simulink model "SMCController1"  (R2018a)
settings: Solver=VariableStepAuto  StartTime=0.0  StopTime=150  RelTol=1e-1
settings Model: Creator=varunpwr  LastModifiedBy=varunpwr

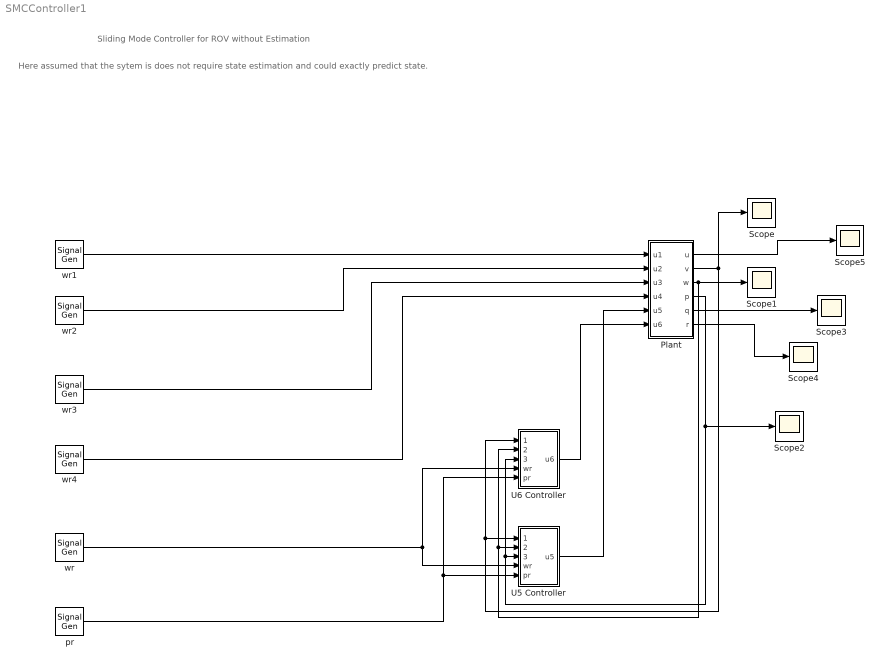
== system SMCController1 ==
  note: Here assumed that the sytem is does not require state estimation and could exactly predict state.
  note: Sliding Mode Controller for ROV without Estimation
  Plant : Subsystem
  Scope{,1..5} (6 alike) : Scope
  U5 Controller : Subsystem
  "U6 Controller " : Subsystem
  pr : SignalGenerator  Amplitude=0  Units=rad/sec
  wr : SignalGenerator  WaveForm=square  Amplitude=0.001  Units=rad/sec
  wr{1..4} (4 alike) : SignalGenerator  Amplitude=0  Units=rad/sec
  wires:
  Plant/2(v) -> Scope/1, "U6 Controller "/1("v var "), U5 Controller/1(v var)
  Plant/3(w) -> Scope1/1, "U6 Controller "/2("w var "), U5 Controller/2("w var ")
  Plant/4(p) -> Scope2/1, "U6 Controller "/3("p var "), U5 Controller/3(p var)
  wr/1 -> U5 Controller/4(wr), "U6 Controller "/4(wr)
  pr/1 -> U5 Controller/5(pr), "U6 Controller "/5(pr)
  U5 Controller/1(u5) -> Plant/5(u5)
  "U6 Controller "/1("u6 ") -> Plant/6(u6)
  wr1/1 -> Plant/1(u1)
  wr2/1 -> Plant/2(u2)
  wr3/1 -> Plant/3(u3)
  wr4/1 -> Plant/4(u4)
  Plant/5(q) -> Scope3/1
  Plant/6(r) -> Scope4/1
  Plant/1("u ") -> Scope5/1

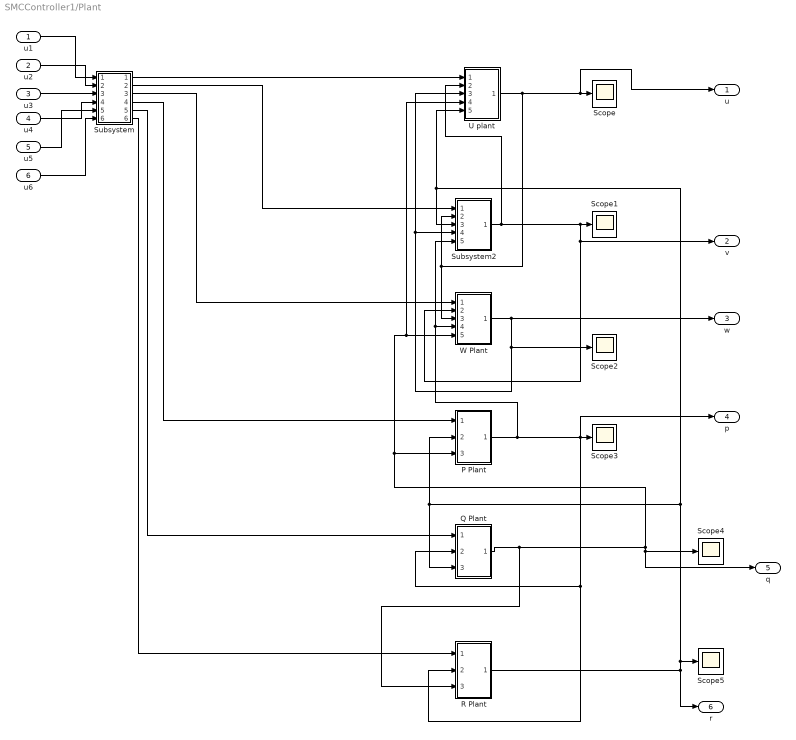
== system SMCController1/Plant ==
  u1 : Inport
  u2 : Inport  Port=2
  u3 : Inport  Port=3
  u4 : Inport  Port=4
  u5 : Inport  Port=5
  u6 : Inport  Port=6
  P Plant : Subsystem
  Q Plant : Subsystem
  "R Plant " : Subsystem
  Scope{,1..5} (6 alike) : Scope
  Subsystem : Subsystem
  Subsystem2 : Subsystem
  "U plant " : Subsystem
  "W Plant " : Subsystem
  "u " : Outport
  v : Outport  Port=2
  w : Outport  Port=3
  p : Outport  Port=4
  q : Outport  Port=5
  r : Outport  Port=6
  wires:
  Subsystem/1(Out1) -> "U plant "/1(In1)
  u2/1 -> Subsystem/2(In2)
  Subsystem/2(Out2) -> Subsystem2/1(In1)
  Subsystem/3(Out3) -> "W Plant "/1(In1)
  u1/1 -> Subsystem/1(In1)
  Q Plant/1(Out1) -> Scope4/1, q/1, P Plant/3("In3 "), "W Plant "/5(In5), "U plant "/4(In4), "R Plant "/3(In3)
  u6/1 -> Subsystem/6(In6)
  Subsystem/6(Out6) -> "R Plant "/1(In1)
  Subsystem2/1(Out1) -> "W Plant "/2(In2), v/1, Scope1/1, "U plant "/2(In2)
  u4/1 -> Subsystem/4(In4)
  "U plant "/1(Out1) -> Subsystem2/2(In2), "W Plant "/3(In3), "u "/1, Scope/1
  u5/1 -> Subsystem/5(In5)
  "R Plant "/1(Out1) -> r/1, Scope5/1, Q Plant/3(In3), P Plant/2(In2), Subsystem2/3(In3), "U plant "/5(In5)
  u3/1 -> Subsystem/3(In3)
  P Plant/1(Out1) -> "R Plant "/2(In2), Q Plant/2(In2), Scope3/1, p/1, "W Plant "/4(In4), Subsystem2/5(In5)
  Subsystem/5(Out5) -> Q Plant/1(In1)
  "W Plant "/1(Out1) -> w/1, Scope2/1, Subsystem2/4(In4), "U plant "/3(In3)
  Subsystem/4(Out4) -> P Plant/1(In1)

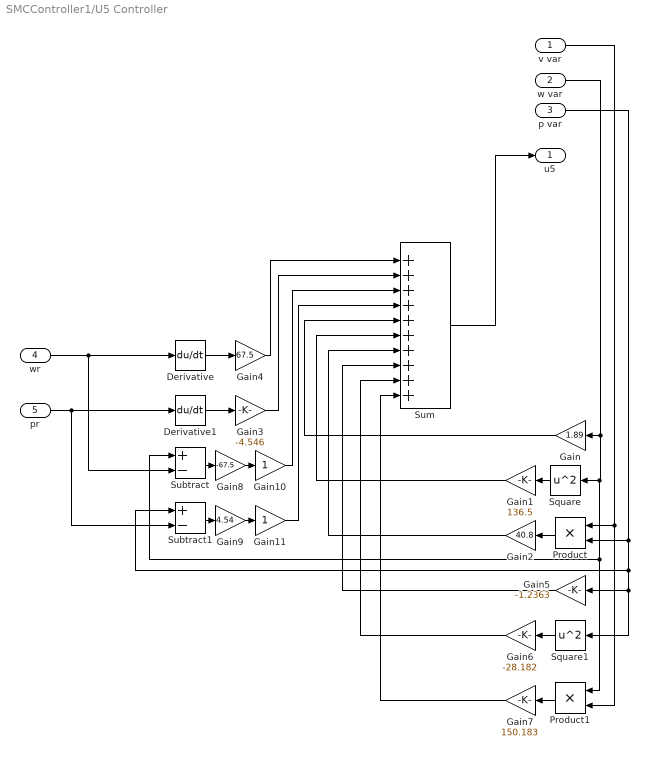
== system SMCController1/U5 Controller ==
  v var : Inport
  "w var " : Inport  Port=2
  p var : Inport  Port=3
  wr : Inport  Port=4
  pr : Inport  Port=5
  Derivative : Derivative
  Derivative1 : Derivative
  Gain : Gain  Gain=1.89
  Gain1 : Gain  Gain=136.5
  Gain10 : Gain
  Gain11 : Gain
  Gain2 : Gain  Gain=40.8
  Gain3 : Gain  Gain=-4.546
  Gain4 : Gain  Gain=67.5
  Gain5 : Gain  Gain=-1.2363
  Gain6 : Gain  Gain=-28.182
  Gain7 : Gain  Gain=150.183
  Gain8 : Gain  Gain=-67.5
  Gain9 : Gain  Gain=4.54
  Product : Product
  Product1 : Product
  Square : Math  Operator=square  SaturateOnIntegerOverflow=on
  Square1 : Math  Operator=square  SaturateOnIntegerOverflow=on
  Subtract : Sum  Inputs=+-
  Subtract1 : Sum  Inputs=+-
  Sum : Sum  Inputs=|++++++++++
  u5 : Outport
  wires:
  Square1/1 -> Gain6/1
  Subtract1/1 -> Gain9/1
  wr/1 -> Subtract/2, Derivative/1
  Gain5/1 -> Sum/8
  "w var "/1 -> Subtract/1, Product1/1, Square/1, Gain/1
  pr/1 -> Subtract1/2, Derivative1/1
  Gain/1 -> Sum/5
  Subtract/1 -> Gain8/1
  v var/1 -> Product1/2, Product/1
  Sum/1 -> u5/1
  p var/1 -> Subtract1/1, Square1/1, Gain5/1, Product/2
  Gain3/1 -> Sum/2
  Square/1 -> Gain1/1
  Gain2/1 -> Sum/7
  Product1/1 -> Gain7/1
  Gain6/1 -> Sum/9
  Gain4/1 -> Sum/1
  Product/1 -> Gain2/1
  Derivative1/1 -> Gain3/1
  Derivative/1 -> Gain4/1
  Gain7/1 -> Sum/10
  Gain1/1 -> Sum/6
  Gain8/1 -> Gain10/1
  Gain10/1 -> Sum/3
  Gain9/1 -> Gain11/1
  Gain11/1 -> Sum/4

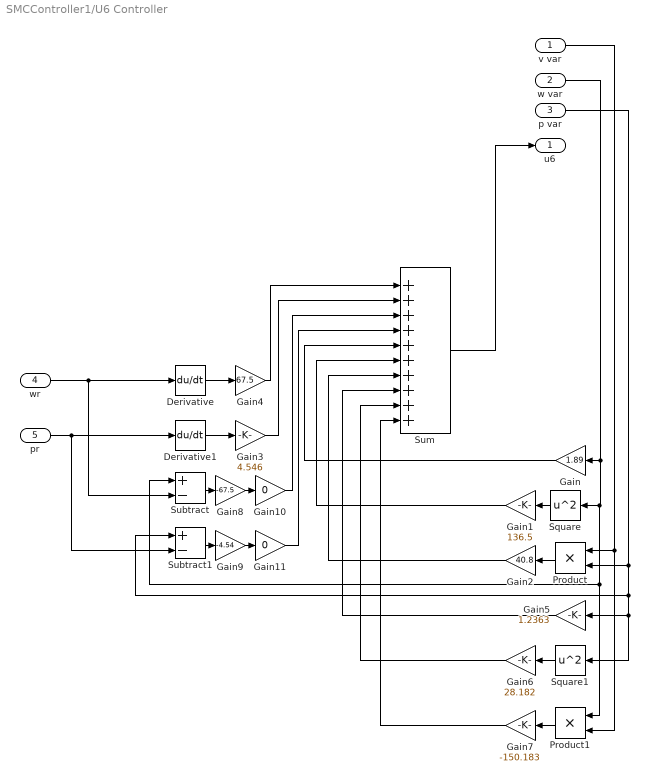
== system SMCController1/U6 Controller  ==
  "v var " : Inport
  "w var " : Inport  Port=2
  "p var " : Inport  Port=3
  wr : Inport  Port=4
  pr : Inport  Port=5
  Derivative : Derivative
  Derivative1 : Derivative
  Gain : Gain  Gain=1.89
  Gain1 : Gain  Gain=136.5
  Gain10 : Gain  Gain=0
  Gain11 : Gain  Gain=0
  Gain2 : Gain  Gain=40.8
  Gain3 : Gain  Gain=4.546
  Gain4 : Gain  Gain=67.5
  Gain5 : Gain  Gain=1.2363
  Gain6 : Gain  Gain=28.182
  Gain7 : Gain  Gain=-150.183
  Gain8 : Gain  Gain=-67.5
  Gain9 : Gain  Gain=-4.54
  Product : Product
  Product1 : Product
  Square : Math  Operator=square  SaturateOnIntegerOverflow=on
  Square1 : Math  Operator=square  SaturateOnIntegerOverflow=on
  Subtract : Sum  Inputs=+-
  Subtract1 : Sum  Inputs=+-
  Sum : Sum  Inputs=|++++++++++
  "u6 " : Outport
  wires:
  Gain1/1 -> Sum/6
  Gain7/1 -> Sum/10
  Derivative/1 -> Gain4/1
  Derivative1/1 -> Gain3/1
  Product/1 -> Gain2/1
  Gain4/1 -> Sum/1
  Gain6/1 -> Sum/9
  Product1/1 -> Gain7/1
  Gain2/1 -> Sum/7
  Square/1 -> Gain1/1
  Gain3/1 -> Sum/2
  "p var "/1 -> Product/2, Gain5/1, Square1/1, Subtract1/1
  Sum/1 -> "u6 "/1
  "v var "/1 -> Product/1, Product1/2
  Subtract/1 -> Gain8/1
  Gain/1 -> Sum/5
  pr/1 -> Derivative1/1, Subtract1/2
  "w var "/1 -> Gain/1, Square/1, Product1/1, Subtract/1
  Gain5/1 -> Sum/8
  wr/1 -> Derivative/1, Subtract/2
  Subtract1/1 -> Gain9/1
  Square1/1 -> Gain6/1
  Gain8/1 -> Gain10/1
  Gain10/1 -> Sum/3
  Gain9/1 -> Gain11/1
  Gain11/1 -> Sum/4

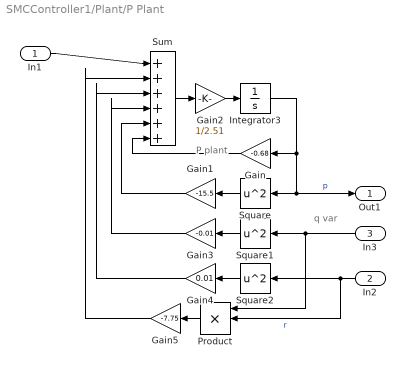
== system SMCController1/Plant/P Plant ==
  note: q var
  note: P plant
  In1 : Inport
  In2 : Inport  Port=2
  "In3 " : Inport  Port=3
  Gain : Gain  Gain=-0.68
  Gain1 : Gain  Gain=-15.5
  Gain2 : Gain  Gain=1/2.51
  Gain3 : Gain  Gain=-0.01
  Gain4 : Gain  Gain=0.01
  Gain5 : Gain  Gain=-7.75
  Integrator3 : Integrator
  Product : Product  Inputs=3
  Square : Math  Operator=square  SaturateOnIntegerOverflow=on
  Square1 : Math  Operator=square  SaturateOnIntegerOverflow=on
  Square2 : Math  Operator=square  SaturateOnIntegerOverflow=on
  Sum : Sum  Inputs=++++|++
  Out1 : Outport
  wires:
  Product/1 -> Gain5/1
  Sum/1 -> Gain2/1
  Gain3/1 -> Sum/4
  Gain4/1 -> Sum/3
  Gain2/1 -> Integrator3/1
  In1/1 -> Sum/1
  Square/1 -> Gain1/1
  Square1/1 -> Gain3/1
  Gain5/1 -> Sum/2
  "In3 "/1 -> Product/1, Square1/1
  Square2/1 -> Gain4/1
  Gain1/1 -> Sum/5
  Gain/1 -> Sum/6
  In2/1 -> Product/2, Square2/1  "r"
  Integrator3/1 -> Out1/1, Square/1, Gain/1  "p"

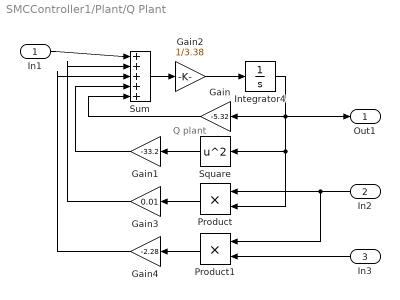
== system SMCController1/Plant/Q Plant ==
  note: Q plant
  In1 : Inport
  In2 : Inport  Port=2
  In3 : Inport  Port=3
  Gain : Gain  Gain=-5.32
  Gain1 : Gain  Gain=-33.2
  Gain2 : Gain  Gain=1/3.38
  Gain3 : Gain  Gain=0.01
  Gain4 : Gain  Gain=-2.28
  Integrator4 : Integrator
  Product : Product
  Product1 : Product
  Square : Math  Operator=square  SaturateOnIntegerOverflow=on
  Sum : Sum  Inputs=+++|++
  Out1 : Outport
  wires:
  Gain1/1 -> Sum/4
  In2/1 -> Product/1, Product1/1
  Gain4/1 -> Sum/3
  In3/1 -> Product1/2
  In1/1 -> Sum/1
  Product/1 -> Gain3/1
  Integrator4/1 -> Out1/1, Square/1, Product/2, Gain/1
  Square/1 -> Gain1/1
  Gain/1 -> Sum/5
  Gain2/1 -> Integrator4/1
  Sum/1 -> Gain2/1
  Product1/1 -> Gain4/1
  Gain3/1 -> Sum/2

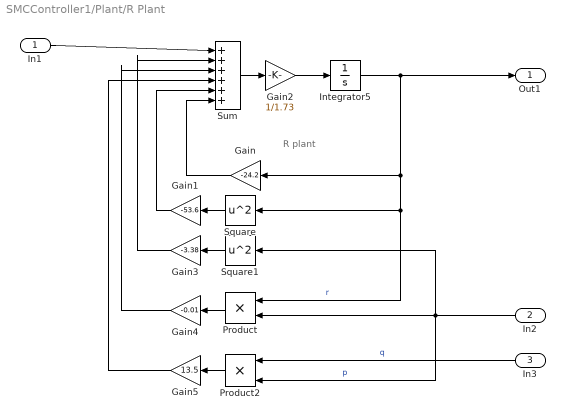
== system SMCController1/Plant/R Plant  ==
  note: R plant
  In1 : Inport
  In2 : Inport  Port=2
  In3 : Inport  Port=3
  Gain : Gain  Gain=-24.2
  Gain1 : Gain  Gain=-53.6
  Gain2 : Gain  Gain=1/1.73
  Gain3 : Gain  Gain=-3.38
  Gain4 : Gain  Gain=-0.01
  Gain5 : Gain  Gain=13.5
  Integrator5 : Integrator
  Product : Product
  Product2 : Product  Inputs=3
  Square : Math  Operator=square  SaturateOnIntegerOverflow=on
  Square1 : Math  Operator=square  SaturateOnIntegerOverflow=on
  Sum : Sum  Inputs=+++|+++
  Out1 : Outport
  wires:
  Product/1 -> Gain4/1
  Gain3/1 -> Sum/2
  Gain4/1 -> Sum/3
  Square/1 -> Gain1/1
  Integrator5/1 -> Product/1, Square/1, Gain/1, Out1/1  "r"
  In2/1 -> Product2/3, Square1/1, Product/2  "p"
  Square1/1 -> Gain3/1
  Gain1/1 -> Sum/5
  In3/1 -> Product2/1  "q"
  Gain/1 -> Sum/6
  Gain2/1 -> Integrator5/1
  Product2/1 -> Gain5/1
  Sum/1 -> Gain2/1
  In1/1 -> Sum/1
  Gain5/1 -> Sum/4

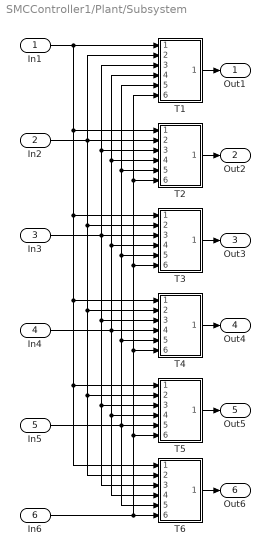
== system SMCController1/Plant/Subsystem ==
  In1 : Inport
  In2 : Inport  Port=2
  In3 : Inport  Port=3
  In4 : Inport  Port=4
  In5 : Inport  Port=5
  In6 : Inport  Port=6
  "T1 " : Subsystem
  T2 : Subsystem
  "T3 " : Subsystem
  T4 : Subsystem
  T5 : Subsystem
  T6 : Subsystem
  Out1 : Outport
  Out2 : Outport  Port=2
  Out3 : Outport  Port=3
  Out4 : Outport  Port=4
  Out5 : Outport  Port=5
  Out6 : Outport  Port=6
  wires:
  "T3 "/1(Out1) -> Out3/1
  "T1 "/1(Out1) -> Out1/1
  T6/1(Out1) -> Out6/1
  T4/1(Out1) -> Out4/1
  In6/1 -> "T1 "/6(In6), T2/6(In6), "T3 "/6(In6), T4/6(In6), T5/6(In6), T6/6(In6)
  T2/1(Out1) -> Out2/1
  T5/1(Out1) -> Out5/1
  In4/1 -> T4/4(In4), T6/4(In4), T5/4(In4), "T3 "/4(In4), T2/4(In4), "T1 "/4(In4)
  In5/1 -> T6/5(In5), T5/5(In5), T4/5(In5), "T3 "/5(In5), T2/5(In5), "T1 "/5(In5)
  In2/1 -> "T3 "/2(In2), T4/2(In2), T5/2(In2), T6/2(In2), T2/2(In2), "T1 "/2(In2)
  In3/1 -> T4/3(In3), T5/3(In3), T6/3(In3), "T3 "/3(In3), "T1 "/3(In3), T2/3(In3)
  In1/1 -> T2/1(In1), "T3 "/1(In1), T4/1(In1), T5/1(In1), T6/1(In1), "T1 "/1(In1)

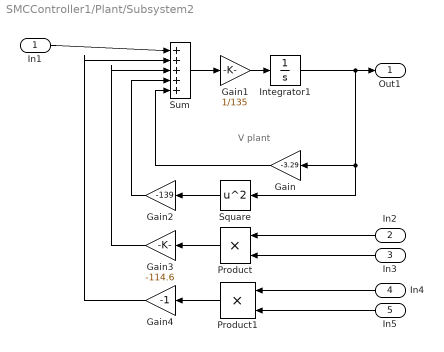
== system SMCController1/Plant/Subsystem2 ==
  note: V plant
  In1 : Inport
  In2 : Inport  Port=2
  In3 : Inport  Port=3
  In4 : Inport  Port=4
  In5 : Inport  Port=5
  Gain : Gain  Gain=-3.29
  Gain1 : Gain  Gain=1/135
  Gain2 : Gain  Gain=-139
  Gain3 : Gain  Gain=-114.6
  Gain4 : Gain  Gain=-1
  Integrator1 : Integrator
  Product : Product
  Product1 : Product
  Square : Math  Operator=square  SaturateOnIntegerOverflow=on
  Sum : Sum  Inputs=+++|++
  Out1 : Outport
  wires:
  Gain2/1 -> Sum/4
  Product/1 -> Gain3/1
  In5/1 -> Product1/2
  In2/1 -> Product/1
  In3/1 -> Product/2
  Integrator1/1 -> Square/1, Gain/1, Out1/1
  In4/1 -> Product1/1
  Gain3/1 -> Sum/3
  Square/1 -> Gain2/1
  Sum/1 -> Gain1/1
  Gain/1 -> Sum/5
  Gain1/1 -> Integrator1/1
  In1/1 -> Sum/1
  Gain4/1 -> Sum/2
  Product1/1 -> Gain4/1

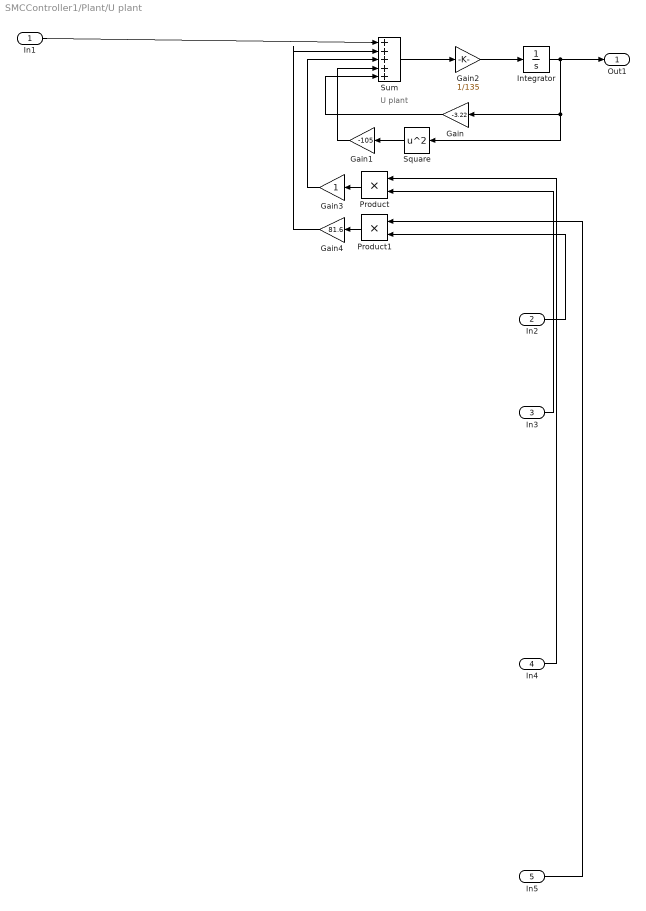
== system SMCController1/Plant/U plant  ==
  note: U plant
  In1 : Inport
  In2 : Inport  Port=2
  In3 : Inport  Port=3
  In4 : Inport  Port=4
  In5 : Inport  Port=5
  Gain : Gain  Gain=-3.22
  Gain1 : Gain  Gain=-105
  Gain2 : Gain  Gain=1/135
  Gain3 : Gain
  Gain4 : Gain  Gain=81.6
  Integrator : Integrator
  Product : Product
  Product1 : Product
  Square : Math  Operator=square  SaturateOnIntegerOverflow=on
  Sum : Sum  Inputs=++|+++
  Out1 : Outport
  wires:
  Gain4/1 -> Sum/2
  In2/1 -> Product1/2
  Sum/1 -> Gain2/1
  In4/1 -> Product/1
  Product/1 -> Gain3/1
  Gain3/1 -> Sum/3
  In5/1 -> Product1/1
  In1/1 -> Sum/1
  Integrator/1 -> Out1/1, Square/1, Gain/1
  Gain2/1 -> Integrator/1
  Product1/1 -> Gain4/1
  In3/1 -> Product/2
  Gain/1 -> Sum/5
  Gain1/1 -> Sum/4
  Square/1 -> Gain1/1

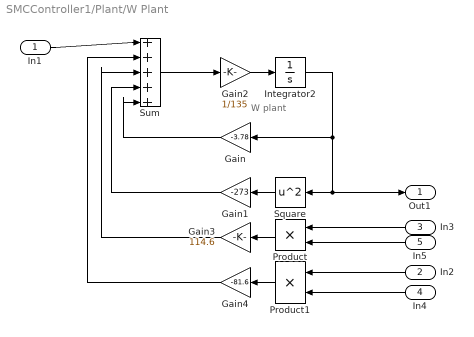
== system SMCController1/Plant/W Plant  ==
  note: W plant
  In1 : Inport
  In2 : Inport  Port=2
  In3 : Inport  Port=3
  In4 : Inport  Port=4
  In5 : Inport  Port=5
  Gain : Gain  Gain=-3.78
  Gain1 : Gain  Gain=-273
  Gain2 : Gain  Gain=1/135
  Gain3 : Gain  Gain=114.6
  Gain4 : Gain  Gain=-81.6
  Integrator2 : Integrator
  Product : Product
  Product1 : Product
  Square : Math  Operator=square  SaturateOnIntegerOverflow=on
  Sum : Sum  Inputs=+++|++
  Out1 : Outport
  wires:
  Gain3/1 -> Sum/3
  Gain/1 -> Sum/5
  Gain1/1 -> Sum/4
  In1/1 -> Sum/1
  Gain2/1 -> Integrator2/1
  Product/1 -> Gain3/1
  In2/1 -> Product1/1
  Integrator2/1 -> Out1/1, Square/1, Gain/1
  Sum/1 -> Gain2/1
  In3/1 -> Product/1
  Product1/1 -> Gain4/1
  Square/1 -> Gain1/1
  Gain4/1 -> Sum/2
  In4/1 -> Product1/2
  In5/1 -> Product/2

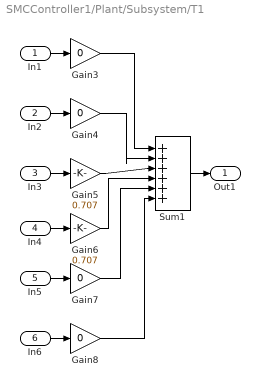
== system SMCController1/Plant/Subsystem/T1  ==
  In1 : Inport
  In2 : Inport  Port=2
  In3 : Inport  Port=3
  In4 : Inport  Port=4
  In5 : Inport  Port=5
  In6 : Inport  Port=6
  Gain{3..4,7..8} (4 alike) : Gain  Gain=0
  Gain5 : Gain  Gain=0.707
  Gain6 : Gain  Gain=0.707
  Sum1 : Sum  Inputs=+|+++++
  Out1 : Outport
  wires:
  Gain6/1 -> Sum1/4
  Sum1/1 -> Out1/1
  Gain4/1 -> Sum1/2
  In6/1 -> Gain8/1
  In3/1 -> Gain5/1
  In2/1 -> Gain4/1
  Gain5/1 -> Sum1/3
  In1/1 -> Gain3/1
  Gain3/1 -> Sum1/1
  In5/1 -> Gain7/1
  Gain7/1 -> Sum1/5
  Gain8/1 -> Sum1/6
  In4/1 -> Gain6/1

== system SMCController1/Plant/Subsystem/T2 ==
  In1 : Inport
  In2 : Inport  Port=2
  In3 : Inport  Port=3
  In4 : Inport  Port=4
  In5 : Inport  Port=5
  In6 : Inport  Port=6
  Gain3 : Gain  Gain=-0.707
  Gain4 : Gain  Gain=0.707
  Gain5 : Gain  Gain=0.707
  Gain6 : Gain  Gain=-0.707
  Gain7 : Gain  Gain=0
  Gain8 : Gain  Gain=0
  Sum1 : Sum  Inputs=+|+++++
  Out1 : Outport
  wires:
  In4/1 -> Gain6/1
  Gain8/1 -> Sum1/6
  Gain7/1 -> Sum1/5
  In5/1 -> Gain7/1
  Gain3/1 -> Sum1/1
  In1/1 -> Gain3/1
  Gain5/1 -> Sum1/3
  In2/1 -> Gain4/1
  In3/1 -> Gain5/1
  In6/1 -> Gain8/1
  Gain4/1 -> Sum1/2
  Sum1/1 -> Out1/1
  Gain6/1 -> Sum1/4

== system SMCController1/Plant/Subsystem/T3  ==
  In1 : Inport
  In2 : Inport  Port=2
  In3 : Inport  Port=3
  In4 : Inport  Port=4
  In5 : Inport  Port=5
  In6 : Inport  Port=6
  Gain3 : Gain  Gain=0.707
  Gain4 : Gain  Gain=0.707
  Gain5 : Gain  Gain=0
  Gain6 : Gain  Gain=0
  Gain7 : Gain
  Gain8 : Gain
  Sum1 : Sum  Inputs=+|+++++
  Out1 : Outport
  wires:
  Gain6/1 -> Sum1/4
  Sum1/1 -> Out1/1
  Gain4/1 -> Sum1/2
  In6/1 -> Gain8/1
  In3/1 -> Gain5/1
  In2/1 -> Gain4/1
  Gain5/1 -> Sum1/3
  In1/1 -> Gain3/1
  Gain3/1 -> Sum1/1
  In5/1 -> Gain7/1
  Gain7/1 -> Sum1/5
  Gain8/1 -> Sum1/6
  In4/1 -> Gain6/1

== system SMCController1/Plant/Subsystem/T4 ==
  In1 : Inport
  In2 : Inport  Port=2
  In3 : Inport  Port=3
  In4 : Inport  Port=4
  In5 : Inport  Port=5
  In6 : Inport  Port=6
  Gain3 : Gain  Gain=0.1099
  Gain4 : Gain  Gain=-0.1099
  Gain5 : Gain  Gain=0
  Gain6 : Gain  Gain=0
  Gain7 : Gain  Gain=-0.275
  Gain8 : Gain  Gain=0.275
  Sum1 : Sum  Inputs=+|+++++
  Out1 : Outport
  wires:
  In4/1 -> Gain6/1
  Gain8/1 -> Sum1/6
  Gain7/1 -> Sum1/5
  In5/1 -> Gain7/1
  Gain3/1 -> Sum1/1
  In1/1 -> Gain3/1
  Gain5/1 -> Sum1/3
  In2/1 -> Gain4/1
  In3/1 -> Gain5/1
  In6/1 -> Gain8/1
  Gain4/1 -> Sum1/2
  Sum1/1 -> Out1/1
  Gain6/1 -> Sum1/4

== system SMCController1/Plant/Subsystem/T5 ==
  In1 : Inport
  In2 : Inport  Port=2
  In3 : Inport  Port=3
  In4 : Inport  Port=4
  In5 : Inport  Port=5
  In6 : Inport  Port=6
  Gain3 : Gain  Gain=0.2789
  Gain4 : Gain  Gain=0.2789
  Gain5 : Gain  Gain=0.3044
  Gain6 : Gain  Gain=0.3044
  Gain7 : Gain  Gain=-0.0355
  Gain8 : Gain  Gain=-0.0355
  Sum1 : Sum  Inputs=+|+++++
  Out1 : Outport
  wires:
  Gain6/1 -> Sum1/4
  Sum1/1 -> Out1/1
  Gain4/1 -> Sum1/2
  In6/1 -> Gain8/1
  In3/1 -> Gain5/1
  In2/1 -> Gain4/1
  Gain5/1 -> Sum1/3
  In1/1 -> Gain3/1
  Gain3/1 -> Sum1/1
  In5/1 -> Gain7/1
  Gain7/1 -> Sum1/5
  Gain8/1 -> Sum1/6
  In4/1 -> Gain6/1

== system SMCController1/Plant/Subsystem/T6 ==
  In1 : Inport
  In2 : Inport  Port=2
  In3 : Inport  Port=3
  In4 : Inport  Port=4
  In5 : Inport  Port=5
  In6 : Inport  Port=6
  Gain3 : Gain  Gain=-0.2789
  Gain4 : Gain  Gain=0.2789
  Gain5 : Gain  Gain=-0.467
  Gain6 : Gain  Gain=0.467
  Gain7 : Gain  Gain=0
  Gain8 : Gain  Gain=0
  Sum1 : Sum  Inputs=+|+++++
  Out1 : Outport
  wires:
  In4/1 -> Gain6/1
  Gain8/1 -> Sum1/6
  Gain7/1 -> Sum1/5
  In5/1 -> Gain7/1
  Gain3/1 -> Sum1/1
  In1/1 -> Gain3/1
  Gain5/1 -> Sum1/3
  In2/1 -> Gain4/1
  In3/1 -> Gain5/1
  In6/1 -> Gain8/1
  Gain4/1 -> Sum1/2
  Sum1/1 -> Out1/1
  Gain6/1 -> Sum1/4
